simulink model "unit_feedback"  (R2023b)
settings: Solver=VariableStepAuto  StartTime=0.0  StopTime=10.0  RelTol=1e-3
values from neighbouring files (symbols this model uses):
  A = sys_d.A    [error_dynamic.m]
  B = sys_d.B    [error_dynamic.m]
  C = sys_d.C    [error_dynamic.m]
  E = Es * Wr    [error_dynamic.m]
  Ts = 0.25    [error_dynamic.m]
  x0 = [0.8;0.2;-0.6;0]    [error_dynamic.m]
settings Model: Creator=Fan Xiuqi  LastModifiedBy=Fan Xiuqi

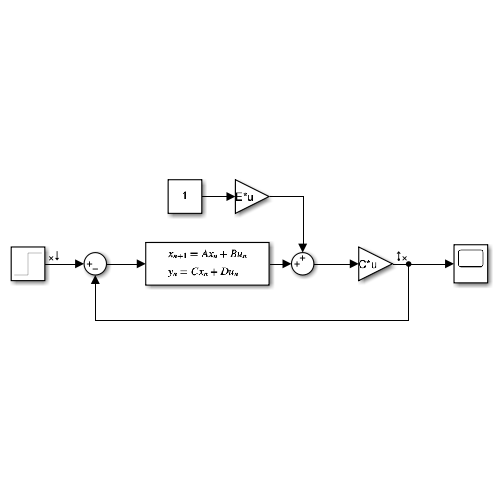
[thumbnail: Simulink's stored preview of the top-level diagram]
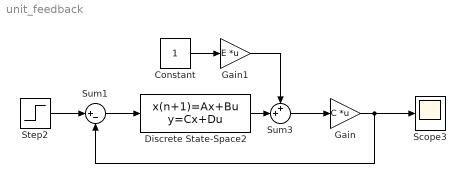
== system unit_feedback ==
  Constant : Constant  SampleTime=Ts
  Discrete State-Space2 : DiscreteStateSpace  A=A  B=B  C=eye(4)  D=zeros(4,1)  InitialCondition=x0  SampleTime=Ts
  Gain : Gain  Gain=C  Multiplication=Matrix(K*u)
  Gain1 : Gain  Gain=E  Multiplication=Matrix(K*u)
  Scope3 : Scope
  Step2 : Step  SampleTime=Ts
  Sum1 : Sum  Inputs=|+-
  Sum3 : Sum  Inputs=++|
  wires:
  Discrete State-Space2/1 -> Sum3/2
  Sum3/1 -> Gain/1
  Step2/1 -> Sum1/1
  Constant/1 -> Gain1/1
  Gain/1 -> Sum1/2, Scope3/1
  Sum1/1 -> Discrete State-Space2/1
  Gain1/1 -> Sum3/1
